simulink model "filtro_sim_fix"  (R2019b)
settings: Solver=ode5  StartTime=0.0  StopTime=0.27  MaxStep=1/512000  RelTol=1e-3  AbsTol=1e-6
undefined symbols (not defined in the file or in its folder): fs
libraries: dspmlti4 x2, dsparch4 x1, dspmisc x1
settings Model: ExtModeTrigMode=oneshot  ExtModeArmWhenConnect=off  ExtModeAutoUpdateStatusClock=off  Creator=The MathWorks, Inc.  LastModifiedBy=luigi
settings SolverCC: AutoScaleAbsTol=off
settings DataIOCC: SaveFormat=Array  SaveOutput=off  SaveTime=off  ReturnWorkspaceOutputs=off  SignalLoggingName=logsOut
settings OptimizationCC: BlockReduction=off  BooleanDataType=off  ExpressionDepthLimit=2147483647  RollThreshold=2  InitFltsAndDblsToZero=on  EfficientMapNaN2IntZero=off  LifeSpan=inf  SimCompilerOptimization=on
settings DebuggingCC: SaveWithParameterizedLinksMsg=none  UnderspecifiedInitializationDetection=Classic  MergeDetectMultiDrivingBlocksExec=none  SignalResolutionControl=TryResolveAllWithWarning  MultiTaskDSMMsg=warning  MultiTaskCondExecSysMsg=none  IntegerOverflowMsg=none  ParameterPrecisionLossMsg=none  FcnCallInpInsideContextMsg=warning  AllowSymbolicDim=off  StateNameClashWarn=warning  SFUnexpectedBacktrackingDiag=warning  SFNoUnconditionalDefaultTransitionDiag=warning  SFExecutionAtInitializationDiag=none  IntegerSaturationMsg=none  ArithmeticOperatorsInVariantConditions=warning
settings HardwareCC: ProdBitPerPointer=32  ProdBitPerSizeT=32  ProdBitPerPtrDiffT=32  ProdLargestAtomicFloat=None  ProdIntDivRoundTo=Undefined  ProdEndianess=Unspecified  ProdWordSize=32  ProdHWDeviceType=32-bit Generic  TargetUnknown=on
settings ModelReferenceCC: PropagateSignalLabelsOutOfModel=off
settings SFSimCC: SimUseLocalCustomCode=off  CustomCodeUndefinedFunction=UseInterfaceOnly
settings RTWCC: RTWUseLocalCustomCode=off
settings CodeAppCC: StateflowObjectComments=on
settings GRTTargetCC: TargetFcnLib=ansi_tfl_tmw.mat  TargetLangStandard=C89/C90 (ANSI)  GeneratePreprocessorConditionals=Disable all  CombineOutputUpdateFcns=off  GRTInterface=on
settings ConfigComp: CovMetricSettings=dw  CovHtmlReporting=on  CovSaveCumulativeToWorkspaceVar=on  CovSaveSingleToWorkspaceVar=on  CovExternalEMLEnable=off

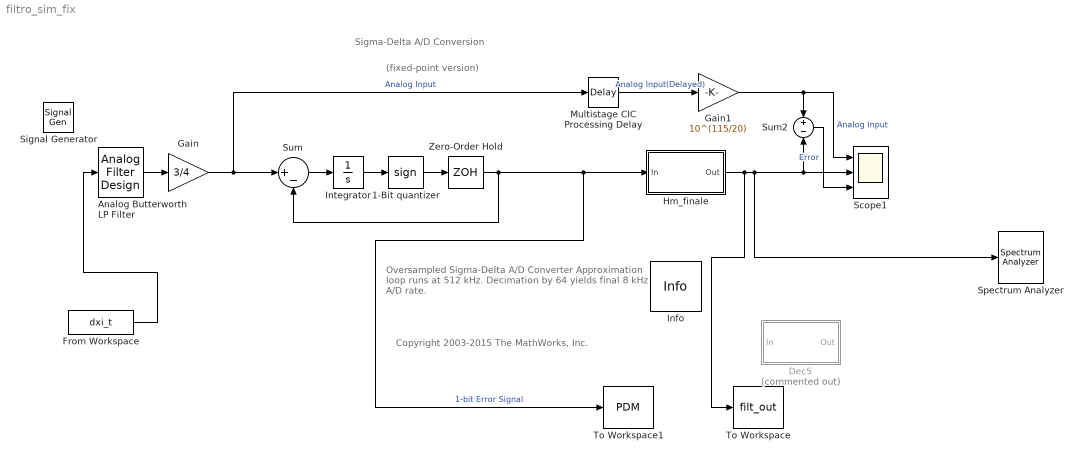
== system filtro_sim_fix ==
  note: Oversampled Sigma-Delta A/D Converter
      | Approximation loop runs at 512 kHz.
      | Decimation by 64 yields final 8 kHz A/D rate.
  note: Sigma-Delta A/D Conversion
  note: (fixed-point version)
  note: Copyright 2003-2015 The MathWorks, Inc.
  1-Bit quantizer : Signum
  Analog Butterworth LP Filter : dsparch4/Analog Filter Design  method=Butterworth  filttype=Lowpass  N=5  Wlo=2*pi*500000  Whi=80  Rp=2  Rs=40
  Dec5 : Subsystem  Tag=BlockMethodSubSystem  Commented=on
  From Workspace : FromWorkspace  VariableName=dxi_t  SampleTime=1/fs
  Gain : Gain  Gain=3/4  SaturateOnIntegerOverflow=on  OutDataTypeStr=Inherit: Same as input  ParamDataTypeStr=Inherit: Same as input
  Gain1 : Gain  Gain=10^(115/20)  SaturateOnIntegerOverflow=on  OutDataTypeStr=Inherit: Same as input  ParamDataTypeStr=Inherit: Same as input
  Hm_finale : Subsystem  Tag=BlockMethodSubSystem
  Info : dspmisc/Info  SystemSampleTime=-1  Latency=0  AutoFrameSizeCalculation=off
      settings: SourceProductName=DSP System Toolbox  SourceProductBaseCode=DS
  Integrator : Integrator
  Multistage CIC Processing Delay : TransportDelay  DelayTime=31/1e6
  Scope1 : Scope  NumInputPorts=3
  Signal Generator : SignalGenerator  Frequency=5000
  Spectrum Analyzer : SpectrumAnalyzer
  Sum : Sum  Inputs=|+-  SaturateOnIntegerOverflow=on  InputSameDT=on  OutDataTypeStr=Inherit: Same as first input
  Sum2 : Sum  Inputs=+-  RndMeth=Nearest  SaturateOnIntegerOverflow=on
  To Workspace : ToWorkspace  VariableName=filt_out  SampleTime=-1
      settings: Save2DSignal=2-D array (concatenate along first dimension)
  To Workspace1 : ToWorkspace  VariableName=PDM  SampleTime=-1
      settings: Save2DSignal=2-D array (concatenate along first dimension)
  Zero-Order Hold : ZeroOrderHold  SampleTime=1/1e6
  wires:
  Zero-Order Hold/1 -> To Workspace1/1, Hm_finale/1(In), Sum/2  "1-bit Error Signal"
  1-Bit quantizer/1 -> Zero-Order Hold/1
  Sum/1 -> Integrator/1
  Integrator/1 -> 1-Bit quantizer/1
  Gain/1 -> Multistage CIC Processing Delay/1, Sum/1  "Analog Input"
  Analog Butterworth LP Filter/1 -> Gain/1
  Sum2/1 -> Scope1/3  "Error"
  Multistage CIC Processing Delay/1 -> Gain1/1  "Analog Input(Delayed)"
  Gain1/1 -> Sum2/1, Scope1/1  "Analog Input"
  Hm_finale/1(Out) -> To Workspace/1, Spectrum Analyzer/1, Sum2/2, Scope1/2
  From Workspace/1 -> Analog Butterworth LP Filter/1

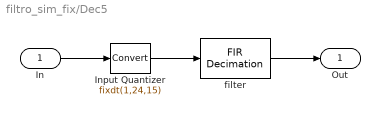
== system filtro_sim_fix/Dec5 ==
  In : Inport
  Input Quantizer : DataTypeConversion  OutDataTypeStr=fixdt(1,24,15)  RndMeth=Round  SaturateOnIntegerOverflow=on
  filter : dspmlti4/FIR Decimation  FilterSource=Dialog parameters  h=[-0.37890625 -1.7734375 -5.54296875 -14.09765625 -31.17578125 -61.97265625 -113.203125 -192.33203125 -306.7421875 -461.828125 -658.72265625 -891.69140625 -1145.20703125 -1391.51953125 -1589.54296875 -1684.6171875 -1611.14453125 -1296.78515625 -669.3515625 334.52734375 1760.16015625 3625.30859375 5912.5546875 8564.37109375 11482.40625 14531.09765625 17546.50390625 20348.95703125 22758.71875 24612.859375 25781.4375 26180.6171875 25781.4375 24612.859375 22758.71875 20348.95703125 17546.50390625 14531.09765625 11482.40625 8564.37109375 5912.5546875 3625.30859375 1760.16015625 334.52734375 -669.3515625 -1296.78515625 -1611.14453125 -1684.6171875 -1589.54296875 -1391.51953125 -1145.20703125 -891.69140625 -658.72265625 -461.828125 -306.7421875 -192.33203125 -113.203125 -61.97265625 -31.17578125 -14.09765625 -5.54296875 -1.7734375 -0.37890625]  D=5  filtStruct=Direct form  FilterObject=FDECIM  framing=Allow multirate processing  inputOffset=0  outputBufInitCond=0  roundingMode=Convergent  overflowMode=off  firstCoeffMode=Binary point scaling  firstCoeffWordLength=24  firstCoeffFracLength=8  firstCoeffDataTypeStr=fixdt(1,24,8)  firstCoeffMin=[]  firstCoeffMax=[]  firstCoeffLastDataTypeStr=fixdt(1,24,8)  prodOutputMode=Binary point scaling  prodOutputWordLength=47  prodOutputFracLength=23  prodOutputDataTypeStr=fixdt(1,47,23)  prodOutputLastDataTypeStr=fixdt(1,47,23)  accumMode=Binary point scaling  accumWordLength=51  accumFracLength=23  accumDataTypeStr=fixdt(1,51,23)  accumLastDataTypeStr=fixdt(1,51,23)  outputMode=Binary point scaling  outputWordLength=51  outputFracLength=23  outputDataTypeStr=fixdt(1,51,23)  outputMin=[]  outputMax=[]  outputLastDataTypeStr=fixdt(1,51,23)
  Out : Outport
  wires:
  In/1 -> Input Quantizer/1
  Input Quantizer/1 -> filter/1
  filter/1 -> Out/1

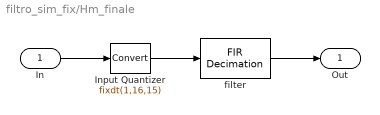
== system filtro_sim_fix/Hm_finale ==
  In : Inport
  Input Quantizer : DataTypeConversion  OutDataTypeStr=fixdt(1,16,15)  RndMeth=Round  SaturateOnIntegerOverflow=on
  filter : dspmlti4/FIR Decimation  FilterSource=Dialog parameters  h=[0.1796875 0.27734375 0.40234375 0.4296875 0.1796875 -0.65234375 -2.52734375 -6.1171875 -12.33984375 -22.3984375 -37.80859375 -60.390625 -92.25390625 -135.72265625 -193.24609375 -267.2421875 -359.88671875 -472.87890625 -607.140625 -762.4921875 -937.30859375 -1128.1796875 -1329.59765625 -1533.6796875 -1730.0078125 -1905.53515625 -2044.66796875 -2129.46484375 -2140.04296875 -2055.140625 -1852.8515625 -1511.515625 -1010.75 -332.546875 537.578125 1609.4765625 2887.32421875 4368.73828125 6044.12109375 7896.23828125 9900.171875 12023.546875 14227.17578125 16466.046875 18690.59765625 20848.34375 22885.66015625 24749.75 26390.62890625 27763.0859375 28828.48828125 29556.375 29925.6953125 29925.6953125 29556.375 28828.48828125 27763.0859375 26390.62890625 24749.75 22885.66015625 20848.34375 18690.59765625 16466.046875 14227.17578125 12023.546875 9900.171875 7896.23828125 6044.12109375 4368.73828125 2887.32421875 1609.4765625 537.578125 -332.546875 -1010.75 -1511.515625 -1852.8515625 -2055.140625 -2140.04296875 -2129.46484375 -2044.66796875 -1905.53515625 -1730.0078125 -1533.6796875 -1329.59765625 -1128.1796875 -937.30859375 -762.4921875 -607.140625 -472.87890625 -359.88671875 -267.2421875 -193.24609375 -135.72265625 -92.25390625 -60.390625 -37.80859375 -22.3984375 -12.33984375 -6.1171875 -2.52734375 -0.65234375 0.1796875 0.4296875 0.40234375 0.27734375 0.1796875]  D=8  filtStruct=Direct form  FilterObject=FDECIM  InputProcessing=Columns as channels (frame based)  framing=Allow multirate processing  inputOffset=0  outputBufInitCond=0  roundingMode=Convergent  overflowMode=off  firstCoeffMode=Binary point scaling  firstCoeffWordLength=28  firstCoeffFracLength=8  firstCoeffDataTypeStr=fixdt(1,28,8)  firstCoeffMin=[]  firstCoeffMax=[]  firstCoeffLastDataTypeStr=fixdt(1,28,8)  prodOutputMode=Binary point scaling  prodOutputWordLength=39  prodOutputFracLength=23  prodOutputDataTypeStr=fixdt(1,39,23)  prodOutputLastDataTypeStr=fixdt(1,39,23)  accumMode=Binary point scaling  accumWordLength=44  accumFracLength=23  accumDataTypeStr=fixdt(1,44,23)  accumLastDataTypeStr=fixdt(1,44,23)  outputMode=Binary point scaling  outputWordLength=44  outputFracLength=23  outputDataTypeStr=fixdt(1,44,23)  outputMin=[]  outputMax=[]  outputLastDataTypeStr=fixdt(1,44,23)
  Out : Outport
  wires:
  In/1 -> Input Quantizer/1
  Input Quantizer/1 -> filter/1
  filter/1 -> Out/1
